simulink model "Model_Simscape_V2"  (R2023a)
settings: Solver=VariableStepAuto  StartTime=0.0  StopTime=10.0  RelTol=1e-3
model workspace (MAT data in the model file):
  Air_density = 1.29
  Body_Temperature = 37
  CtrlData_Max = 100
  CtrlData_Min = 0
  Detpress_to_Vavle.detpress = [1.45 1.55 1.6 1.65 1.7 1.75 1.8 1.85 1.9 1.95 2 2.05 5 7 26 42 60 78 99 112]
  Detpress_to_Vavle.vavle = [0.999 0.94 0.89 0.84 0.78 0.73 0.68 0.63 0.57 0.52 0.47 0.42 0.36 0.31 0.25 0.21 0.15 0.1 0.05 0]
  E_respriatory = 10
  ExpValve.opening_vector = [0 0.052 0.105 0.157 0.21 0.263 0.315 0.368 0.421 0.473 0.526 0.578 0.631 0.684 0.736 0.789 0.842 0.894 0.947 1]
  ExpValve.Cv_vector = [0.0001 0.81 1.114 1.723 3.218 3.547 4.603 5.2063 6.069 6.57 6.974 7.226 7.563 7.856 7.997 8.565 8.84 9.267 9.621 10.487]
  ExpValve.threshold = 0.0011
  ExpValve.zerovalue = 0
  ExpValve.Cross_Area = 0.000314159265359
  ExpValve.fullValue = 1
  FRC = 2
  Fan.shaftspeed = [14400 15600 16800 18000 19200 20400 21600 22800 24000 25200 26400 27600 28800 30000 31200 32400 33600 34800 36000 37200 38400 39600 40800 42000 43200 44400 45600 46800 48000]
  Fan.presstable = [0; 1; 2; 3; 4; 5; 6; 7; 8]
  Fan.flowvector = [97.5714285714 106 114 122 128.666666667 137 147.5 160.272727273 169.5 178.424242424 186.909090909 195.25 ... (261 elements, 29x9)]
  Fan.efficiency = [0.45  0.45  NaN  NaN  NaN  NaN  NaN  NaN  NaN; 0.45  0.45  NaN  NaN  NaN  NaN  NaN  NaN  NaN; 0.45  0.45  NaN  NaN  NaN  NaN  NaN  NaN  NaN; 0.45  0.45  NaN  NaN  NaN  NaN  NaN  NaN  NaN; 0.45  0.45  NaN  NaN  NaN  NaN  NaN  NaN  NaN; 0.45  0.45  NaN  NaN  NaN  NaN  NaN  NaN  NaN; 0.45  0.45  0.45  NaN  NaN  NaN  NaN  NaN  NaN; 0.45  0.45  0.45  NaN  NaN  NaN  NaN  NaN  NaN; 0.45  0.45  0.45  0.45  NaN  NaN  NaN  NaN  NaN; 0.45  0.45  0.45  0.45  NaN  NaN  NaN  NaN  NaN; 0.45  0.45  0.45  0.45  NaN  NaN  NaN  NaN  NaN; 0.45  0.45  0.45  0.45  NaN  NaN  NaN  NaN  NaN; 0.45  0.45  0.45  0.45  NaN  NaN  NaN  NaN  NaN; 0.45  0.45  0.45  0.45  0.45  NaN  NaN  NaN  NaN; 0.45  0.45  0.45  0.45  0.45  NaN  NaN  NaN  NaN; 0.45  0.45  0.45  0.45  0.45  NaN  NaN  NaN  NaN; 0.45  0.45  0.45  0.45  0.45  0.45  NaN  NaN  NaN; 0.45  0.45  0.45  0.45  0.45  0.45  NaN  NaN  NaN; 0.45  0.45  0.45  0.45  0.45  0.45  0.45  NaN  NaN; 0.45  0.45  0.45  0.45  0.45  0.45  0.45  NaN  NaN; 0.45  0.45  0.45  0.45  0.45  0.45  0.45  NaN  NaN; 0.45  0.45  0.45  0.45  0.45  0.45  0.45  NaN  NaN; 0.45  0.45  0.45  0.45  0.45  0.45  0.45  0.45  NaN; 0.45  0.45  0.45  0.45  0.45  0.45  0.45  0.45  NaN; 0.45  0.45  0.45  0.45  0.45  0.45  0.45  0.45  NaN; 0.45  0.45  0.45  0.45  0.45  0.45  0.45  0.45  0.45; 0.45  0.45  0.45  0.45  0.45  0.45  0.45  0.45  0.45; 0.45  0.45  0.45  0.45  0.45  0.45  0.45  0.45  0.45; 0.45  0.45  0.45  0.45  0.45  0.45  0.45  0.45  0.45]
  Fan.Inlerarea_A = 0.000314159265359
  Fan.Inlerarea_B = 0.000314159265359
  Flow_Resistance_1.resistance = 0.1
  Flow_Resistance_1.pressure_drop = 0.1
  Flow_Resistance_1.flow_rate = 1
  Flow_Resistance_1.Crosss_Area = 0.000314159265359
  Flow_Resistance_2.resistance = 0.1
  Flow_Resistance_2.pressure_drop = 0.1
  Flow_Resistance_2.flow_rate = 1
  Flow_Resistance_2.Crosss_Area = 0.000314159265359
  Hard_Stop.Lower_bound = -1e-06
  InspValve.opening_vector = [0 0.052 0.105 0.157 0.21 0.263 0.315 0.368 0.421 0.473 0.526 0.578 0.631 0.684 0.736 0.789 0.842 0.894 0.947 1]
  InspValve.Cv_vector = [0.0001 0.81 1.114 1.723 3.218 3.547 4.603 5.2063 6.069 6.57 6.974 7.226 7.563 7.856 7.997 8.565 8.84 9.267 9.621 10.487]
  InspValve.threshold = 0.0011
  InspValve.zerovalue = 0
  InspValve.Cross_Area = 0.000314159265359
  L_to_m3 = 0.001
  Mask.Chamber_volume = 0.0002
  Mask.A_area = 0.000314159265359
  Mask.B_area = 0.000314159265359
  Mask.C_area = 0.000314159265359
  Pa_to_cmH2O = 0.0101974428892
  Percent_to_Unit = 0.01
  Pipe_1.r = 0.01
  Pipe_1.longlength = 0.1
  Pipe_1.area = 0.000314159265359
  Pipe_1.diameter = 0.02
  Pipe_2.r = 0.01
  Pipe_2.longlength = 0.1
  Pipe_2.area = 0.000314159265359
  Pipe_2.diameter = 0.02
  Pipe_3.r = 0.01
  Pipe_3.longlength = 0.1
  Pipe_3.area = 0.000314159265359
  Pipe_3.diameter = 0.02
  R_respiratory = 2
  Reservoir.Cross_area = 0.000314159265359
  Trachea.Pipe_length = 0.15
  Trachea.area = 0.000314159265359
  Trachea.Hydraulic_diameter = 0.02
  Volume_Max = 0.9
  cmH2O_to_Pa = 98.0638
  cmH2O_to_kPa = 0.0981
  lung.Interface_area = 1
  lung.Dead_volume = 1e-06
  lung.Cross_area = 0.000314159265359
  percentage_to_rpm = 600
libraries: fl_lib x62, nesl_utility x13, SimscapeFluids_lib x3, aerolibatmos2 x1
(part 1 of 3)
settings Model: DataDictionary=MVEPP_DataDict.sldd  Creator=xuluyu  LastModifiedBy=xuluyu
settings OptimizationCC: UseDivisionForNetSlopeComputation=on

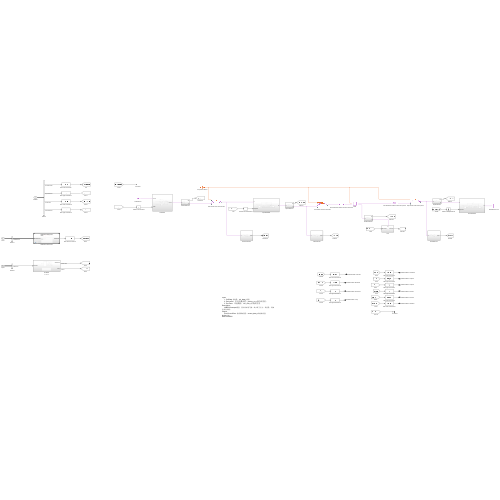
[thumbnail: Simulink's stored preview of the top-level diagram]
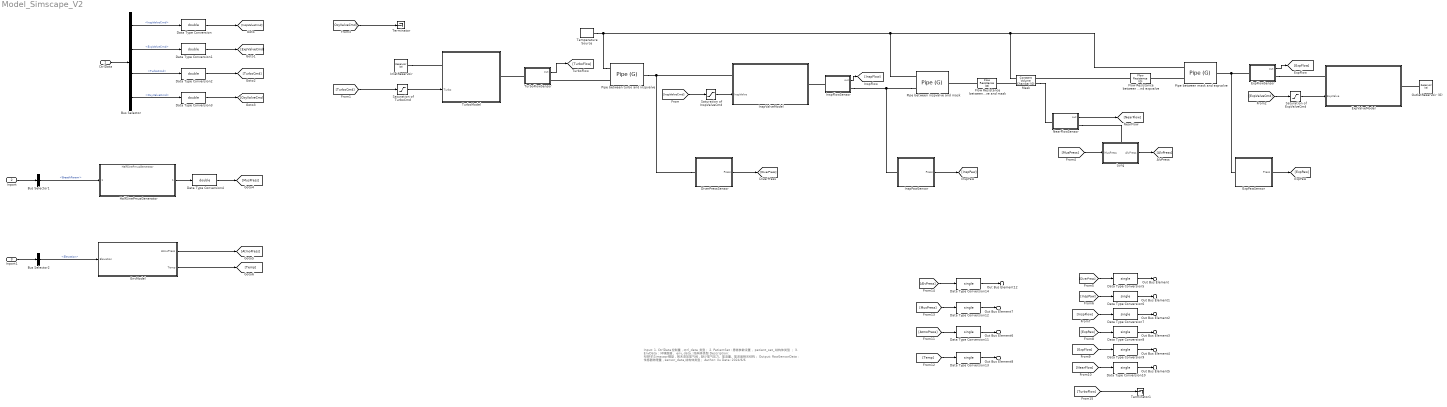
== system Model_Simscape_V2 ==
  note: Input:
      | 1. CtrlData: 控制量，ctrl_data_t类型；
      | 2. PatientSet ：患者参数设置， patient_set_t 结构体类型 ；
      | 3. EnvData ：环境数据， env_data_t 结构体类型
      | Description:
      | NIBP的Simscape模型，暂未添加氧气阀，缺少氧气压力、氧流量、氧浓度相关结构；
      | Output:
      | RawSensorData : 传感器物理量，sensor_data_t结构体类型；
      | Author: Xu
      | Data: 2024/6/6
  CtrlData : Inport  OutDataTypeStr=Bus: ctrl_data_t
  Inport : Inport  Port=2  OutDataTypeStr=Bus: patient_set_t
  Inport1 : Inport  Port=3  OutDataTypeStr=Bus: env_data_t
  Bus Selector : BusSelector  OutputSignals=InspValveCmd,ExpValveCmd,TurboCmd,OxyValveCmd
  Bus Selector1 : BusSelector  OutputSignals=BreathParam
  Bus Selector2 : BusSelector  OutputSignals=Elevation
  Data Type Conversion{,1..4} (5 alike) : DataTypeConversion  OutDataTypeStr=double  SaturateOnIntegerOverflow=off  RndMeth=Floor
  Data Type Conversion{5..14} (10 alike) : DataTypeConversion  OutDataTypeStr=single  SaturateOnIntegerOverflow=off  RndMeth=Floor
  DiverPressSensor : Subsystem
  EnvModel : Subsystem  Description=环境模型
      settings: AttributesFormatString=%<Description>
  ExpFlowSensor : Subsystem
  ExpPawSensor : Subsystem
  ExpValveModel : Subsystem
      settings: PortSchema="{\"entries\":[{\"content\":{\"sides\":[{\"content\":{\"connectorIds\":[\"LConn1\",\"In1\"]},\"type\":\"ConnectorPlacement.EquallySpacedRectSide\",\"uuid\":\"c1491169-4dad-48f4-8472-367eebf90c5f\"},{\"content\":{\"connectorIds\":[\"RConn1\"],\"side\":\"RIGHT\"},\"type\":\"ConnectorPlacement.EquallySpacedRectSide\",\"uuid\":\"0545f3b4-3593-4e73-91f2-3a40a520eda3\"},{\"content\":{\"side\":\"TOP\"},\"type\":\"ConnectorPlacement.EquallySpacedRectSide\",\"uuid\":\"424c4b06-b659-46bd-af11-3177a58fa4cf\"}]},\"type\":\"ConnectorPlacement.EquallySpacedConnector\",\"uuid\":\"6932a250-8b99-4db1-8a9b-8eee5e551d75\"}],\"packageUris\":[\"http://schema.mathworks.com/mf0/Connector/R2020b\"],\"version\":\"1.0\"}"
  Flow Resistance between inspvalve and mask : fl_lib/Gas/Elements/Flow Resistance (G)  delta_p_nominal=Flow_Resistance_1.pressure_drop*cmH2O_to_kPa kPa  mdot_nominal=Flow_Resistance_1.flow_rate*L_to_m3*Air_density kg/s  rho_nominal=0 kg/m^3  area=Flow_Resistance_1.Crosss_Area m^2  laminar_fraction=1e-3
      settings: InternalSimscapePortConfiguration="{\"Bottom\":[],\"Left\":[{\"id\":\"A\",\"label\":\"A\",\"type\":\"foundation.gas.gas\"}],\"Right\":[{\"id\":\"B\",\"label\":\"B\",\"type\":\"foundation.gas.gas\"}],\"Top\":[]}"
  Flow Resistance between mask and expvalve : fl_lib/Gas/Elements/Flow Resistance (G)  delta_p_nominal=Flow_Resistance_2.pressure_drop*cmH2O_to_kPa kPa  mdot_nominal=Flow_Resistance_2.flow_rate*L_to_m3*Air_density kg/s  rho_nominal=0 kg/m^3  area=Flow_Resistance_2.Crosss_Area m^2  laminar_fraction=1e-3
      settings: InternalSimscapePortConfiguration="{\"Bottom\":[],\"Left\":[{\"id\":\"A\",\"label\":\"A\",\"type\":\"foundation.gas.gas\"}],\"Right\":[{\"id\":\"B\",\"label\":\"B\",\"type\":\"foundation.gas.gas\"}],\"Top\":[]}"
  HalfSinePmusGenerator : ModelReference  ModelNameDialog=HalfSinePmusGenerator.slx  SimulationMode=Normal  ModelReferenceVersion=1.36
  InletReservoir : fl_lib/Gas/Elements/Reservoir (G)  pressure_spec=foundation.enum.pressure_spec.atmospheric  reservoir_pressure=0.101325 MPa  reservoir_temperature=293.15 K  area_A=Reservoir.Cross_area m^2
  "InspFlowSensor " : Subsystem
  InspPawSensor : Subsystem
  InspValveModel : Subsystem
      settings: PortSchema="{\"entries\":[{\"content\":{\"sides\":[{\"content\":{\"connectorIds\":[\"LConn1\",\"In1\"]},\"type\":\"ConnectorPlacement.EquallySpacedRectSide\",\"uuid\":\"c1491169-4dad-48f4-8472-367eebf90c5f\"},{\"content\":{\"connectorIds\":[\"RConn1\"],\"side\":\"RIGHT\"},\"type\":\"ConnectorPlacement.EquallySpacedRectSide\",\"uuid\":\"0545f3b4-3593-4e73-91f2-3a40a520eda3\"},{\"content\":{\"side\":\"TOP\"},\"type\":\"ConnectorPlacement.EquallySpacedRectSide\",\"uuid\":\"424c4b06-b659-46bd-af11-3177a58fa4cf\"}]},\"type\":\"ConnectorPlacement.EquallySpacedConnector\",\"uuid\":\"6932a250-8b99-4db1-8a9b-8eee5e551d75\"}],\"packageUris\":[\"http://schema.mathworks.com/mf0/Connector/R2020b\"],\"version\":\"1.0\"}"
  Lung : Subsystem
      settings: PortSchema="{\"entries\":[{\"content\":{\"sides\":[{\"content\":{\"connectorIds\":[\"In1\"]},\"type\":\"ConnectorPlacement.EquallySpacedRectSide\",\"uuid\":\"62194df3-39be-42c9-91e0-55317383e8ff\"},{\"content\":{\"connectorIds\":[\"Out1\"],\"side\":\"RIGHT\"},\"type\":\"ConnectorPlacement.EquallySpacedRectSide\",\"uuid\":\"0a91156d-be32-4862-8ff5-ef7fbd9fceb6\"},{\"content\":{\"connectorIds\":[\"LConn1\"],\"side\":\"TOP\"},\"type\":\"ConnectorPlacement.EquallySpacedRectSide\",\"uuid\":\"74941641-d695-41de-be65-3ac62a0b8891\"}]},\"type\":\"ConnectorPlacement.EquallySpacedConnector\",\"uuid\":\"a19a4056-8f95-4fbc-822a-a9438a1c1a7f\"}],\"packageUris\":[\"http://schema.mathworks.com/mf0/Connector/R2020b\"],\"version\":\"1.0\"}"
  Mask : fl_lib/Gas/Elements/Constant Volume Chamber (G)  volume=Mask.Chamber_volume m^3  num_ports=foundation.enum.num_ports.three  area_A=Mask.A_area m^2  area_B=Mask.B_area m^2  area_C=Mask.C_area m^2  area_D=0.01 m^2  p_I_specify=off  p_I_priority=High  p_I=0.101325 MPa  p_I_nominal_specify=off  p_I_nominal_unit=MPa  p_I_nominal_value=1  T_I_specify=off  T_I_priority=High  T_I=37 degC  T_I_nominal_specify=off  T_I_nominal_unit=K  T_I_nominal_value=1  rho_I_specify=off  rho_I_priority=None  rho_I=1.2 kg/m^3  rho_I_nominal_specify=off  rho_I_nominal_unit=kg/m^3  rho_I_nominal_value=1
      settings: InternalSimscapePortConfiguration="{\"Bottom\":[],\"Left\":[{\"id\":\"A\",\"label\":\"A\",\"type\":\"foundation.gas.gas\"},{\"id\":\"H\",\"label\":\"H\",\"type\":\"foundation.thermal.thermal\"}],\"Right\":[{\"id\":\"B\",\"label\":\"B\",\"type\":\"foundation.gas.gas\"},{\"id\":\"C\",\"label\":\"C\",\"type\":\"foundation.gas.gas\"}],\"Top\":[]}"
  "NearFlowSensor " : Subsystem
  OutletReservoir (G) : fl_lib/Gas/Elements/Reservoir (G)  pressure_spec=foundation.enum.pressure_spec.atmospheric  reservoir_pressure=0.101325 MPa  reservoir_temperature=293.15 K  area_A=Reservoir.Cross_area m^2
  Pipe between inspvalve and mask : fl_lib/Gas/Elements/Pipe (G)  length=Pipe_2.longlength m  area=Pipe_2.area m^2  Dh=Pipe_2.diameter m  length_add=0.1 m  roughness=15e-6 m  Re_lam=2000  Re_tur=4000  shape_factor=64  Nu_lam=3.66  p_I_specify=off  p_I_priority=High  p_I=0.101325 MPa  p_I_nominal_specify=off  p_I_nominal_unit=MPa  p_I_nominal_value=1  T_I_specify=off  T_I_priority=High  T_I=293.15 K  T_I_nominal_specify=off  T_I_nominal_unit=K  T_I_nominal_value=1  rho_I_specify=off  rho_I_priority=None  rho_I=1.2 kg/m^3  rho_I_nominal_specify=off  rho_I_nominal_unit=kg/m^3  rho_I_nominal_value=1
  Pipe between mask and expvalve : fl_lib/Gas/Elements/Pipe (G)  length=Pipe_3.longlength m  area=Pipe_3.area m^2  Dh=Pipe_3.diameter m  length_add=0.1 m  roughness=15e-6 m  Re_lam=2000  Re_tur=4000  shape_factor=64  Nu_lam=3.66  p_I_specify=off  p_I_priority=High  p_I=0.101325 MPa  p_I_nominal_specify=off  p_I_nominal_unit=MPa  p_I_nominal_value=1  T_I_specify=off  T_I_priority=High  T_I=293.15 K  T_I_nominal_specify=off  T_I_nominal_unit=K  T_I_nominal_value=1  rho_I_specify=off  rho_I_priority=None  rho_I=1.2 kg/m^3  rho_I_nominal_specify=off  rho_I_nominal_unit=kg/m^3  rho_I_nominal_value=1
  Pipe between turbo and inspvalve : fl_lib/Gas/Elements/Pipe (G)  length=Pipe_1.longlength m  area=Pipe_1.area m^2  Dh=Pipe_1.diameter m  length_add=0.1 m  roughness=15e-6 m  Re_lam=2000  Re_tur=4000  shape_factor=64  Nu_lam=3.66  p_I_specify=on  p_I_priority=High  p_I=0.101325 MPa  p_I_nominal_specify=off  p_I_nominal_unit=MPa  p_I_nominal_value=1  T_I_specify=on  T_I_priority=High  T_I=293.15 K  T_I_nominal_specify=off  T_I_nominal_unit=K  T_I_nominal_value=1  rho_I_specify=off  rho_I_priority=None  rho_I=1.2 kg/m^3  rho_I_nominal_specify=off  rho_I_nominal_unit=kg/m^3  rho_I_nominal_value=1
  Saturation of ExpValveCmd : Saturate  UpperLimit=CtrlData_Max  LowerLimit=CtrlData_Min
  Saturation of InspValveCmd : Saturate  UpperLimit=CtrlData_Max  LowerLimit=CtrlData_Min
  Saturation of TurboCmd : Saturate  UpperLimit=CtrlData_Max  LowerLimit=CtrlData_Min
  Temperature Source : fl_lib/Thermal/Thermal Sources/Temperature Source  temperature=293.15 K
  Terminator : Terminator
  Terminator1 : Terminator
  TurboFlowSensor : Subsystem
  TurboModel : Subsystem
      settings: PortSchema="{\"entries\":[{\"content\":{\"sides\":[{\"content\":{\"connectorIds\":[\"LConn1\",\"In1\"]},\"type\":\"ConnectorPlacement.EquallySpacedRectSide\",\"uuid\":\"c1491169-4dad-48f4-8472-367eebf90c5f\"},{\"content\":{\"connectorIds\":[\"RConn1\"],\"side\":\"RIGHT\"},\"type\":\"ConnectorPlacement.EquallySpacedRectSide\",\"uuid\":\"0545f3b4-3593-4e73-91f2-3a40a520eda3\"},{\"content\":{\"side\":\"TOP\"},\"type\":\"ConnectorPlacement.EquallySpacedRectSide\",\"uuid\":\"424c4b06-b659-46bd-af11-3177a58fa4cf\"}]},\"type\":\"ConnectorPlacement.EquallySpacedConnector\",\"uuid\":\"6932a250-8b99-4db1-8a9b-8eee5e551d75\"}],\"packageUris\":[\"http://schema.mathworks.com/mf0/Connector/R2020b\"],\"version\":\"1.0\"}"
  Out Bus Element6 : Outport  PortName=RawSensorData  Element=AtomPress
  Out Bus Element12 : Outport  PortName=RawSensorData  Element=AlvPress
  Out Bus Element7 : Outport  PortName=RawSensorData  Element=MusPress
  Out Bus Element2 : Outport  PortName=RawSensorData  Element=InspFlow
  Out Bus Element4 : Outport  PortName=RawSensorData  Element=ExpFlow
  Out Bus Element5 : Outport  PortName=RawSensorData  Element=NearFlow
  Out Bus Element1 : Outport  PortName=RawSensorData  Element=InspPaw
  Out Bus Element3 : Outport  PortName=RawSensorData  Element=ExpPaw
  Out Bus Element : Outport  PortName=RawSensorData  Element=DrivePress
  Out Bus Element8 : Outport  PortName=RawSensorData  Element=Temp
  wires:
  ExpFlowSensor/1(out) -> [ExpFlow]
  TurboFlowSensor/1(out) -> [TurboFlow]
  "NearFlowSensor "/1(out) -> [NearFlow]
  "InspFlowSensor "/1(out) -> [InspFlow]
  InspPawSensor/1(Press) -> [InspPaw]
  DiverPressSensor/1(Press) -> [DiverPress]
  ExpPawSensor/1(Press) -> [ExpPaw]
  CtrlData/1 -> Bus Selector/1
  Bus Selector/1 -> Data Type Conversion/1  "<InspValveCmd>"
  Bus Selector/2 -> Data Type Conversion1/1  "<ExpValveCmd>"
  Bus Selector/3 -> Data Type Conversion2/1  "<TurboCmd>"
  Bus Selector/4 -> Data Type Conversion3/1  "<OxyValveCmd>"
  Saturation of TurboCmd/1 -> TurboModel/1(Turbo)
  [TurboCmd] -> Saturation of TurboCmd/1
  Saturation of InspValveCmd/1 -> InspValveModel/1(InspValve)
  [InspValveCmd] -> Saturation of InspValveCmd/1
  [ExpValveCmd] -> Saturation of ExpValveCmd/1
  Saturation of ExpValveCmd/1 -> ExpValveModel/1(ExpValve)
  [OxyValveCmd] -> Terminator/1
  HalfSinePmusGenerator/1 -> Data Type Conversion4/1
  [MusPress] -> Lung/1(MusPress)
  Inport/1 -> Bus Selector1/1
  Bus Selector1/1 -> HalfSinePmusGenerator/1  "<BreathParam>"
  Data Type Conversion/1 -> [InspValveCmd]
  Data Type Conversion1/1 -> [ExpValveCmd]
  Data Type Conversion2/1 -> [TurboCmd]
  Data Type Conversion3/1 -> [OxyValveCmd]
  Data Type Conversion4/1 -> [MusPress]
  Inport1/1 -> Bus Selector2/1
  Bus Selector2/1 -> EnvModel/1(Elevation)  "<Elevation>"
  EnvModel/1(AtmoPress) -> [AtmoPress]
  EnvModel/2(Temp) -> [Temp]
  Lung/1(AlvPress) -> [AlvPress]
  [DiverPress] -> Data Type Conversion5/1
  [InspPaw] -> Data Type Conversion6/1
  [InspFlow] -> Data Type Conversion7/1
  [ExpPaw] -> Data Type Conversion8/1
  [ExpFlow] -> Data Type Conversion9/1
  [NearFlow] -> Data Type Conversion10/1
  [AtmoPress] -> Data Type Conversion11/1
  [MusPress] -> Data Type Conversion12/1
  [Temp] -> Data Type Conversion13/1
  Data Type Conversion5/1 -> Out Bus Element/1
  Data Type Conversion6/1 -> Out Bus Element1/1
  Data Type Conversion7/1 -> Out Bus Element2/1
  Data Type Conversion8/1 -> Out Bus Element3/1
  Data Type Conversion9/1 -> Out Bus Element4/1
  Data Type Conversion10/1 -> Out Bus Element5/1
  Data Type Conversion11/1 -> Out Bus Element6/1
  Data Type Conversion12/1 -> Out Bus Element7/1
  Data Type Conversion13/1 -> Out Bus Element8/1
  [AlvPress] -> Data Type Conversion14/1
  Data Type Conversion14/1 -> Out Bus Element12/1
  [TurboFlow] -> Terminator1/1
  connections:
  Pipe between mask and expvalve/RConn1 -- ExpFlowSensor/LConn1 -- ExpPawSensor/LConn1
  Pipe between inspvalve and mask/LConn1 -- "InspFlowSensor "/RConn1 -- InspPawSensor/LConn1
  DiverPressSensor/LConn1 -- InspValveModel/LConn1 -- Pipe between turbo and inspvalve/RConn1
  Pipe between turbo and inspvalve/LConn2 -- Pipe between mask and expvalve/LConn2 -- Mask/LConn2 -- Pipe between inspvalve and mask/LConn2 -- Temperature Source/LConn1
  Flow Resistance between inspvalve and mask/LConn1 -- Pipe between inspvalve and mask/RConn1
  "NearFlowSensor "/RConn1 -- Lung/LConn1
  Flow Resistance between mask and expvalve/LConn1 -- Mask/RConn2
  OutletReservoir (G)/LConn1 -- ExpValveModel/RConn1
  TurboFlowSensor/LConn1 -- TurboModel/RConn1
  ExpFlowSensor/RConn1 -- ExpValveModel/LConn1
  InletReservoir/LConn1 -- TurboModel/LConn1
  Mask/LConn1 -- Flow Resistance between inspvalve and mask/RConn1
  Pipe between turbo and inspvalve/LConn1 -- TurboFlowSensor/RConn1
  Mask/RConn1 -- "NearFlowSensor "/LConn1
  Pipe between mask and expvalve/LConn1 -- Flow Resistance between mask and expvalve/RConn1
  "InspFlowSensor "/LConn1 -- InspValveModel/RConn1

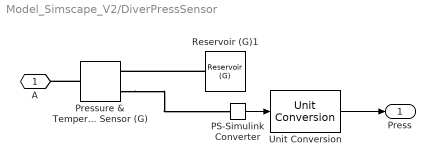
== system Model_Simscape_V2/DiverPressSensor ==
  PS-Simulink Converter : nesl_utility/PS-Simulink Converter  PhysicalDomain=network_engine_domain  SubClassName=ps_output  LeftPortType=input  RightPortType=output  PseudoPeriodic=off  Frequencies=[]  VectorFormat=inherit  Unit=Pa  AffineConversion=off
  Pressure & Temperature Sensor (G) : fl_lib/Gas/Sensors/Pressure & Temperature Sensor (G)  reference=foundation.enum.MeasurementReference.difference  pressure=true  pressure_spec=foundation.enum.PressureMeasementSpec.Absolute  temperature=false
      settings: InternalSimscapePortConfiguration="{\"Bottom\":[],\"Left\":[{\"id\":\"A\",\"label\":\"A\",\"type\":\"foundation.gas.gas\"}],\"Right\":[{\"id\":\"B\",\"label\":\"B\",\"type\":\"foundation.gas.gas\"},{\"id\":\"P\",\"label\":\"P\",\"type\":\"output\"}],\"Top\":[]}"
  Reservoir (G)1 : fl_lib/Gas/Elements/Reservoir (G)  pressure_spec=foundation.enum.pressure_spec.atmospheric  reservoir_pressure=0.101325 MPa  reservoir_temperature=293.15 K  area_A=Reservoir.Cross_area m^2
  Unit Conversion : UnitConversion
  A : PMIOPort  Side=Left
  Press : Outport  Unit=hPa
  wires:
  PS-Simulink Converter/1 -> Unit Conversion/1
  Unit Conversion/1 -> Press/1
  connections:
  Reservoir (G)1/LConn1 -- Pressure & Temperature Sensor (G)/RConn1
  Pressure & Temperature Sensor (G)/LConn1 -- A/RConn1
  Pressure & Temperature Sensor (G)/RConn2 -- PS-Simulink Converter/LConn1

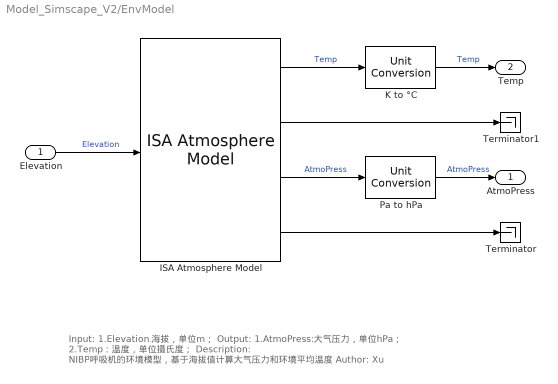
== system Model_Simscape_V2/EnvModel ==
  note: Input:
      | 	1.Elevation:海拔，单位m；
      | Output:
      | 	1.AtmoPress:大气压力，单位hPa；
      | 	2.Temp：温度，单位摄氏度；
      | Description:
      | 	NIBP呼吸机的环境模型，基于海拔值计算大气压力和环境平均温度
      | Author:
      | 	Xu
  Elevation : Inport  OutDataTypeStr=int16  Unit=m
  ISA Atmosphere Model : aerolibatmos2/ISA Atmosphere Model  custom=off  g=9.80665  gamma=1.4  R=287.0531  L=0.0065  h_trop=11000  h_strat=20000  rho0=1.225  P0=101325  T0=288.15  h0=0
  K to °C : UnitConversion  OutputType=Inherit: Inherit via back propagation
  Pa to hPa : UnitConversion  OutputType=Inherit: Inherit via back propagation
  Terminator : Terminator
  Terminator1 : Terminator
  AtmoPress : Outport  OutDataTypeStr=single  Unit=hPa
  Temp : Outport  Port=2  OutDataTypeStr=single  Unit=°C
  wires:
  Elevation/1 -> ISA Atmosphere Model/1  "Elevation"
  Pa to hPa/1 -> AtmoPress/1  "AtmoPress"
  ISA Atmosphere Model/4 -> Terminator/1
  K to °C/1 -> Temp/1  "Temp"
  ISA Atmosphere Model/2 -> Terminator1/1
  ISA Atmosphere Model/3 -> Pa to hPa/1  "AtmoPress"
  ISA Atmosphere Model/1 -> K to °C/1  "Temp"

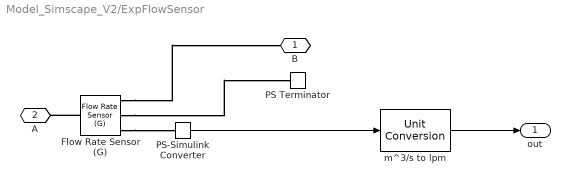
== system Model_Simscape_V2/ExpFlowSensor ==
  Flow Rate Sensor (G) : fl_lib/Gas/Sensors/Flow Rate Sensor (G)  mass_flow_measure=true  volumetric_flow_measure=true  volumetric_flow_conditions=foundation.enum.volumetric_flow_conditions.actual  p_std=0.101325 MPa  T_std=20 degC  energy_flow_measure=false
      settings: InternalSimscapePortConfiguration="{\"Bottom\":[],\"Left\":[{\"id\":\"A\",\"label\":\"A\",\"type\":\"foundation.gas.gas\"}],\"Right\":[{\"id\":\"B\",\"label\":\"B\",\"type\":\"foundation.gas.gas\"},{\"id\":\"M\",\"label\":\"M\",\"type\":\"output\"},{\"id\":\"V\",\"label\":\"V\",\"type\":\"output\"}],\"Top\":[]}"
  PS Terminator : fl_lib/Physical Signals/Sinks/PS Terminator
  PS-Simulink Converter : nesl_utility/PS-Simulink Converter  PhysicalDomain=network_engine_domain  SubClassName=ps_output  LeftPortType=input  RightPortType=output  PseudoPeriodic=off  Frequencies=[]  VectorFormat=inherit  Unit=m^3/s  AffineConversion=off
  m^3/s to lpm : UnitConversion
  B : PMIOPort  Side=Right
  A : PMIOPort  Port=2  Side=Left
  out : Outport  Unit=lpm
  wires:
  PS-Simulink Converter/1 -> m^3/s to lpm/1
  m^3/s to lpm/1 -> out/1
  connections:
  Flow Rate Sensor (G)/RConn1 -- B/RConn1
  Flow Rate Sensor (G)/LConn1 -- A/RConn1
  Flow Rate Sensor (G)/RConn2 -- PS Terminator/LConn1
  Flow Rate Sensor (G)/RConn3 -- PS-Simulink Converter/LConn1

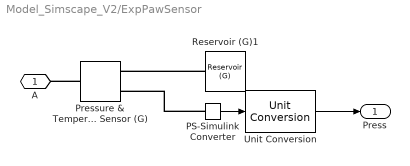
== system Model_Simscape_V2/ExpPawSensor ==
  PS-Simulink Converter : nesl_utility/PS-Simulink Converter  PhysicalDomain=network_engine_domain  SubClassName=ps_output  LeftPortType=input  RightPortType=output  PseudoPeriodic=off  Frequencies=[]  VectorFormat=inherit  Unit=inherit  AffineConversion=off
  Pressure & Temperature Sensor (G) : fl_lib/Gas/Sensors/Pressure & Temperature Sensor (G)  reference=foundation.enum.MeasurementReference.difference  pressure=true  pressure_spec=foundation.enum.PressureMeasementSpec.Absolute  temperature=false
      settings: InternalSimscapePortConfiguration="{\"Bottom\":[],\"Left\":[{\"id\":\"A\",\"label\":\"A\",\"type\":\"foundation.gas.gas\"}],\"Right\":[{\"id\":\"B\",\"label\":\"B\",\"type\":\"foundation.gas.gas\"},{\"id\":\"P\",\"label\":\"P\",\"type\":\"output\"}],\"Top\":[]}"
  Reservoir (G)1 : fl_lib/Gas/Elements/Reservoir (G)  pressure_spec=foundation.enum.pressure_spec.atmospheric  reservoir_pressure=0.101325 MPa  reservoir_temperature=293.15 K  area_A=Reservoir.Cross_area m^2
  Unit Conversion : UnitConversion
  A : PMIOPort  Side=Left
  Press : Outport  Unit=hPa
  wires:
  PS-Simulink Converter/1 -> Unit Conversion/1
  Unit Conversion/1 -> Press/1
  connections:
  PS-Simulink Converter/LConn1 -- Pressure & Temperature Sensor (G)/RConn2
  Reservoir (G)1/LConn1 -- Pressure & Temperature Sensor (G)/RConn1
  Pressure & Temperature Sensor (G)/LConn1 -- A/RConn1

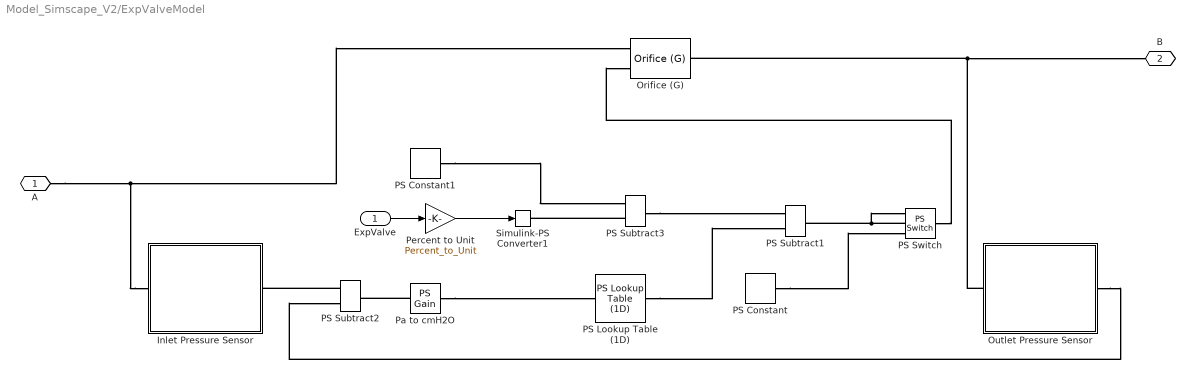
== system Model_Simscape_V2/ExpValveModel ==
  ExpValve : Inport
  " Inlet Pressure Sensor" : Subsystem
  " Outlet Pressure Sensor" : Subsystem
  Orifice (G) : SimscapeFluids_lib/Gas/Valves & Orifices/Orifice (G)  orifice_type=foundation.enum.constant_variable.variable  orifice_parameterization=fluids.gas.valves_orifices.enum.OrificeParameterization.Cv  opening_characteristic=fluids.gas.valves_orifices.enum.OpeningCharacteristics.Tabulated  Cv_constant=4  Cv_max=4  L_Cv_TLU=ExpValve.opening_vector  Cv_TLU=ExpValve.Cv_vector  xT_Cv=0.7  Kv_constant=3.6  Kv_max=3.6  L_Kv_TLU=0 : 0.2 : 1  Kv_TLU=[1e-06, .72, 1.44, 2.16, 2.88, 3.6]  xT_Kv=0.7  C_constant=12 l/(bar*s)  B_crit_constant=0.3  C_max=12 l/(bar*s)  B_crit_linear=0.3  L_C_TLU=0 : 0.2 : 1  C_TLU=[1e-05, 2.4, 4.8, 7.2, 9.6, 12] l/(bar*s)  B_crit_TLU=0.3 * ones(1, 6)  m=0.5  T_ref_C=293.15 K  rho_ref_C=1.185 kg/m^3  orifice_area_constant=1e-4 m^2  orifice_area_max=1e-4 m^2  L_orifice_area_TLU=0 : 0.2 : 1  orifice_area_TLU=[1e-10, 2e-05, 4e-05, 6e-05, 8e-05, .0001] m^2  Cd=0.64  leakage_fraction=1e-6  smoothing_factor=0.01  B_lam=0.999  area=ExpValve.Cross_Area m^2
      settings: InternalSimscapePortConfiguration="{\"Bottom\":[],\"Left\":[{\"id\":\"A\",\"label\":\"A\",\"type\":\"foundation.gas.gas\"},{\"id\":\"L\",\"label\":\"L\",\"type\":\"input\"}],\"Right\":[{\"id\":\"B\",\"label\":\"B\",\"type\":\"foundation.gas.gas\"}],\"Top\":[]}"
  PS Constant : fl_lib/Physical Signals/Sources/PS Constant  constant=ExpValve.zerovalue
  PS Constant1 : fl_lib/Physical Signals/Sources/PS Constant  constant=ExpValve.fullValue
  PS Lookup Table (1D) : fl_lib/Physical Signals/Lookup Tables/PS Lookup Table (1D)  x=Detpress_to_Vavle.detpress  f=Detpress_to_Vavle.vavle  interp_method=simscape.enum.interpolation.linear  extrap_method=simscape.enum.extrapolation.nearest
  PS Subtract1 : fl_lib/Physical Signals/Functions/PS Subtract
  PS Subtract2 : fl_lib/Physical Signals/Functions/PS Subtract
  PS Subtract3 : fl_lib/Physical Signals/Functions/PS Subtract
  PS Switch : fl_lib/Physical Signals/Nonlinear Operators/PS Switch  Threshold=ExpValve.threshold
      settings: InternalSimscapePortConfiguration="{\"Bottom\":[],\"Left\":[{\"id\":\"I1\",\"label\":\"\",\"type\":\"input\"},{\"id\":\"I2\",\"label\":\"\",\"type\":\"input\"},{\"id\":\"I3\",\"label\":\"\",\"type\":\"input\"}],\"Right\":[{\"id\":\"O\",\"label\":\"\",\"type\":\"output\"}],\"Top\":[]}"
  Pa to cmH2O : fl_lib/Physical Signals/Functions/PS Gain  gain=Pa_to_cmH2O 1/Pa
  Percent to Unit : Gain  Gain=Percent_to_Unit
  Simulink-PS Converter1 : nesl_utility/Simulink-PS Converter  PhysicalDomain=network_engine_domain  SubClassName=ps_input  LeftPortType=input  RightPortType=output  PseudoPeriodic=off  Frequencies=[]  NoiseDistribution=none  NoiseParameters=[]  Unit=1  AffineConversion=off  FilteringAndDerivatives=provide  SimscapeFilterOrder=1  InputFilterTimeConstant=0.001  UdotUserProvided=0
  A : PMIOPort  Side=Left
  B : PMIOPort  Port=2  Side=Right
  wires:
  Percent to Unit/1 -> Simulink-PS Converter1/1
  ExpValve/1 -> Percent to Unit/1
  connections:
  " Outlet Pressure Sensor"/LConn1 -- Orifice (G)/RConn1 -- B/RConn1
  PS Subtract2/LConn1 -- " Inlet Pressure Sensor"/RConn1
  PS Constant/RConn1 -- PS Switch/LConn3
  PS Switch/LConn2 -- PS Switch/LConn1 -- PS Subtract1/RConn1
  PS Lookup Table (1D)/RConn1 -- PS Subtract1/LConn2
  " Outlet Pressure Sensor"/RConn1 -- PS Subtract2/LConn2
  " Inlet Pressure Sensor"/LConn1 -- Orifice (G)/LConn1 -- A/RConn1
  PS Switch/RConn1 -- Orifice (G)/LConn2
  Pa to cmH2O/LConn1 -- PS Subtract2/RConn1
  Pa to cmH2O/RConn1 -- PS Lookup Table (1D)/LConn1
  PS Subtract3/LConn2 -- Simulink-PS Converter1/RConn1
  PS Subtract3/RConn1 -- PS Subtract1/LConn1
  PS Constant1/RConn1 -- PS Subtract3/LConn1

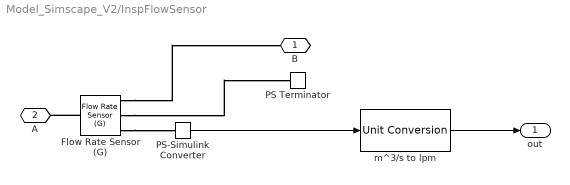
== system Model_Simscape_V2/InspFlowSensor  ==
  Flow Rate Sensor (G) : fl_lib/Gas/Sensors/Flow Rate Sensor (G)  mass_flow_measure=true  volumetric_flow_measure=true  volumetric_flow_conditions=foundation.enum.volumetric_flow_conditions.actual  p_std=0.101325 MPa  T_std=20 degC  energy_flow_measure=false
      settings: InternalSimscapePortConfiguration="{\"Bottom\":[],\"Left\":[{\"id\":\"A\",\"label\":\"A\",\"type\":\"foundation.gas.gas\"}],\"Right\":[{\"id\":\"B\",\"label\":\"B\",\"type\":\"foundation.gas.gas\"},{\"id\":\"M\",\"label\":\"M\",\"type\":\"output\"},{\"id\":\"V\",\"label\":\"V\",\"type\":\"output\"}],\"Top\":[]}"
  PS Terminator : fl_lib/Physical Signals/Sinks/PS Terminator
  PS-Simulink Converter : nesl_utility/PS-Simulink Converter  PhysicalDomain=network_engine_domain  SubClassName=ps_output  LeftPortType=input  RightPortType=output  PseudoPeriodic=off  Frequencies=[]  VectorFormat=inherit  Unit=m^3/s  AffineConversion=off
  m^3/s to lpm : UnitConversion
  B : PMIOPort  Side=Right
  A : PMIOPort  Port=2  Side=Left
  out : Outport  Unit=lpm
  wires:
  PS-Simulink Converter/1 -> m^3/s to lpm/1
  m^3/s to lpm/1 -> out/1
  connections:
  Flow Rate Sensor (G)/RConn1 -- B/RConn1
  Flow Rate Sensor (G)/LConn1 -- A/RConn1
  Flow Rate Sensor (G)/RConn2 -- PS Terminator/LConn1
  Flow Rate Sensor (G)/RConn3 -- PS-Simulink Converter/LConn1

== system Model_Simscape_V2/InspPawSensor ==
  PS-Simulink Converter : nesl_utility/PS-Simulink Converter  PhysicalDomain=network_engine_domain  SubClassName=ps_output  LeftPortType=input  RightPortType=output  PseudoPeriodic=off  Frequencies=[]  VectorFormat=inherit  Unit=inherit  AffineConversion=off
  Pressure & Temperature Sensor (G) : fl_lib/Gas/Sensors/Pressure & Temperature Sensor (G)  reference=foundation.enum.MeasurementReference.difference  pressure=true  pressure_spec=foundation.enum.PressureMeasementSpec.Absolute  temperature=false
      settings: InternalSimscapePortConfiguration="{\"Bottom\":[],\"Left\":[{\"id\":\"A\",\"label\":\"A\",\"type\":\"foundation.gas.gas\"}],\"Right\":[{\"id\":\"B\",\"label\":\"B\",\"type\":\"foundation.gas.gas\"},{\"id\":\"P\",\"label\":\"P\",\"type\":\"output\"}],\"Top\":[]}"
  Reservoir (G)1 : fl_lib/Gas/Elements/Reservoir (G)  pressure_spec=foundation.enum.pressure_spec.atmospheric  reservoir_pressure=0.101325 MPa  reservoir_temperature=293.15 K  area_A=Reservoir.Cross_area m^2
  Unit Conversion : UnitConversion
  A : PMIOPort  Side=Left
  Press : Outport  Unit=hPa
  wires:
  PS-Simulink Converter/1 -> Unit Conversion/1
  Unit Conversion/1 -> Press/1
  connections:
  Pressure & Temperature Sensor (G)/LConn1 -- A/RConn1
  Reservoir (G)1/LConn1 -- Pressure & Temperature Sensor (G)/RConn1
  PS-Simulink Converter/LConn1 -- Pressure & Temperature Sensor (G)/RConn2

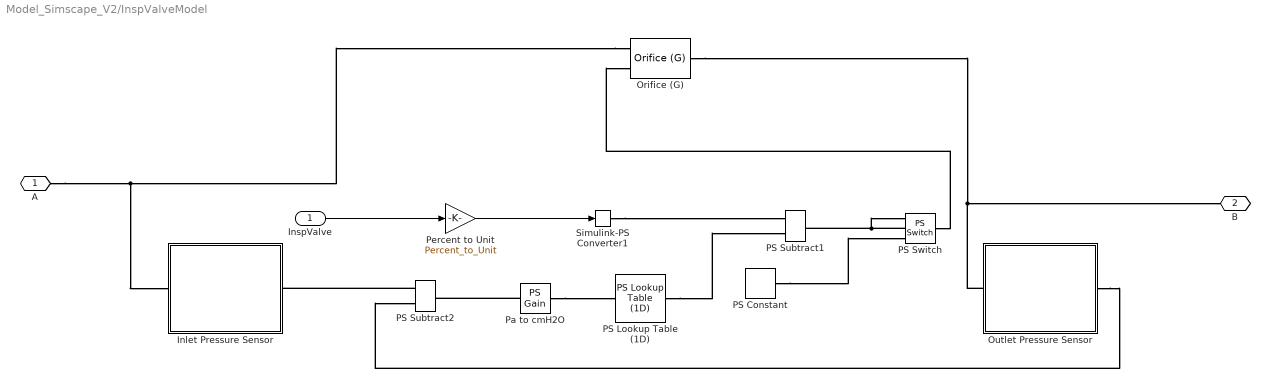
== system Model_Simscape_V2/InspValveModel ==
  InspValve : Inport
  " Inlet Pressure Sensor" : Subsystem
  " Outlet Pressure Sensor" : Subsystem
  Orifice (G) : SimscapeFluids_lib/Gas/Valves & Orifices/Orifice (G)  orifice_type=foundation.enum.constant_variable.variable  orifice_parameterization=fluids.gas.valves_orifices.enum.OrificeParameterization.Cv  opening_characteristic=fluids.gas.valves_orifices.enum.OpeningCharacteristics.Tabulated  Cv_constant=4  Cv_max=4  L_Cv_TLU=InspValve.opening_vector  Cv_TLU=InspValve.Cv_vector  xT_Cv=0.7  Kv_constant=3.6  Kv_max=3.6  L_Kv_TLU=0 : 0.2 : 1  Kv_TLU=[1e-06, .72, 1.44, 2.16, 2.88, 3.6]  xT_Kv=0.7  C_constant=12 l/(bar*s)  B_crit_constant=0.3  C_max=12 l/(bar*s)  B_crit_linear=0.3  L_C_TLU=0 : 0.2 : 1  C_TLU=[1e-05, 2.4, 4.8, 7.2, 9.6, 12] l/(bar*s)  B_crit_TLU=0.3 * ones(1, 6)  m=0.5  T_ref_C=293.15 K  rho_ref_C=1.185 kg/m^3  orifice_area_constant=1e-4 m^2  orifice_area_max=1e-4 m^2  L_orifice_area_TLU=0 : 0.2 : 1  orifice_area_TLU=[1e-10, 2e-05, 4e-05, 6e-05, 8e-05, .0001] m^2  Cd=0.64  leakage_fraction=1e-6  smoothing_factor=0.01  B_lam=0.999  area=InspValve.Cross_Area m^2
      settings: InternalSimscapePortConfiguration="{\"Bottom\":[],\"Left\":[{\"id\":\"A\",\"label\":\"A\",\"type\":\"foundation.gas.gas\"},{\"id\":\"L\",\"label\":\"L\",\"type\":\"input\"}],\"Right\":[{\"id\":\"B\",\"label\":\"B\",\"type\":\"foundation.gas.gas\"}],\"Top\":[]}"
  PS Constant : fl_lib/Physical Signals/Sources/PS Constant  constant=InspValve.zerovalue
  PS Lookup Table (1D) : fl_lib/Physical Signals/Lookup Tables/PS Lookup Table (1D)  x=Detpress_to_Vavle.detpress  f=Detpress_to_Vavle.vavle  interp_method=simscape.enum.interpolation.linear  extrap_method=simscape.enum.extrapolation.nearest
  PS Subtract1 : fl_lib/Physical Signals/Functions/PS Subtract
  PS Subtract2 : fl_lib/Physical Signals/Functions/PS Subtract
  PS Switch : fl_lib/Physical Signals/Nonlinear Operators/PS Switch  Threshold=InspValve.threshold
      settings: InternalSimscapePortConfiguration="{\"Bottom\":[],\"Left\":[{\"id\":\"I1\",\"label\":\"\",\"type\":\"input\"},{\"id\":\"I2\",\"label\":\"\",\"type\":\"input\"},{\"id\":\"I3\",\"label\":\"\",\"type\":\"input\"}],\"Right\":[{\"id\":\"O\",\"label\":\"\",\"type\":\"output\"}],\"Top\":[]}"
  Pa to cmH2O : fl_lib/Physical Signals/Functions/PS Gain  gain=Pa_to_cmH2O 1/Pa
  Percent to Unit : Gain  Gain=Percent_to_Unit
  Simulink-PS Converter1 : nesl_utility/Simulink-PS Converter  PhysicalDomain=network_engine_domain  SubClassName=ps_input  LeftPortType=input  RightPortType=output  PseudoPeriodic=off  Frequencies=[]  NoiseDistribution=none  NoiseParameters=[]  Unit=1  AffineConversion=off  FilteringAndDerivatives=provide  SimscapeFilterOrder=1  InputFilterTimeConstant=0.001  UdotUserProvided=0
  A : PMIOPort  Side=Left
  B : PMIOPort  Port=2  Side=Right
  wires:
  InspValve/1 -> Percent to Unit/1
  Percent to Unit/1 -> Simulink-PS Converter1/1
  connections:
  Orifice (G)/RConn1 -- " Outlet Pressure Sensor"/LConn1 -- B/RConn1
  PS Subtract2/LConn1 -- " Inlet Pressure Sensor"/RConn1
  PS Constant/RConn1 -- PS Switch/LConn3
  PS Switch/LConn2 -- PS Subtract1/RConn1 -- PS Switch/LConn1
  PS Lookup Table (1D)/RConn1 -- PS Subtract1/LConn2
  " Outlet Pressure Sensor"/RConn1 -- PS Subtract2/LConn2
  Orifice (G)/LConn1 -- A/RConn1 -- " Inlet Pressure Sensor"/LConn1
  Simulink-PS Converter1/RConn1 -- PS Subtract1/LConn1
  PS Switch/RConn1 -- Orifice (G)/LConn2
  Pa to cmH2O/LConn1 -- PS Subtract2/RConn1
  Pa to cmH2O/RConn1 -- PS Lookup Table (1D)/LConn1

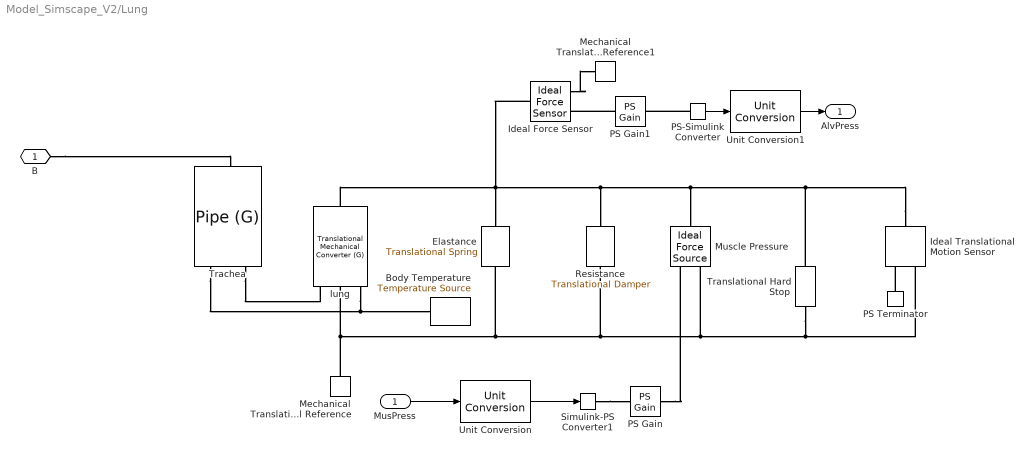
== system Model_Simscape_V2/Lung ==
  MusPress : Inport  Unit=hPa
  Body Temperature : fl_lib/Thermal/Thermal Sources/Temperature Source  temperature="Body_Temperature  degC"
  Elastance : fl_lib/Mechanical/Translational Elements/Translational Spring  spr_rate=E_respriatory*(lung.Interface_area^2)*(cmH2O_to_Pa/L_to_m3) N/m  v_specify=off  v_priority=None  v=0 m/s  v_nominal_specify=off  v_nominal_unit=m/s  v_nominal_value=1  f_specify=off  f_priority=None  f=0 N  f_nominal_specify=off  f_nominal_unit=N  f_nominal_value=1  x_specify=off  x_priority=High  x=0 m  x_nominal_specify=off  x_nominal_unit=m  x_nominal_value=1
  Ideal Force Sensor : fl_lib/Mechanical/Mechanical Sensors/Ideal Force Sensor
  Ideal Translational Motion Sensor : fl_lib/Mechanical/Mechanical Sensors/Ideal Translational Motion Sensor  reference=foundation.enum.MeasurementReference.difference  acceleration_port=false  velocity_port=false  position_port=true  offset=FRC*L_to_m3 m
      settings: InternalSimscapePortConfiguration="{\"Bottom\":[],\"Left\":[{\"id\":\"R\",\"label\":\"R\",\"type\":\"foundation.mechanical.translational.translational\"}],\"Right\":[{\"id\":\"C\",\"label\":\"C\",\"type\":\"foundation.mechanical.translational.translational\"},{\"id\":\"P\",\"label\":\"P\",\"type\":\"output\"}],\"Top\":[]}"
  Mechanical Translational Reference : fl_lib/Mechanical/Translational Elements/Mechanical Translational Reference
  Mechanical Translational Reference1 : fl_lib/Mechanical/Translational Elements/Mechanical Translational Reference
  Muscle Pressure : fl_lib/Mechanical/Mechanical Sources/Ideal Force Source
  PS Gain : fl_lib/Physical Signals/Functions/PS Gain  gain=lung.Interface_area m^2
  PS Gain1 : fl_lib/Physical Signals/Functions/PS Gain  gain=1/lung.Interface_area 1/m^2
  PS Terminator : fl_lib/Physical Signals/Sinks/PS Terminator
  PS-Simulink Converter : nesl_utility/PS-Simulink Converter  PhysicalDomain=network_engine_domain  SubClassName=ps_output  LeftPortType=input  RightPortType=output  PseudoPeriodic=off  Frequencies=[]  VectorFormat=inherit  Unit=Pa  AffineConversion=off
  Resistance : fl_lib/Mechanical/Translational Elements/Translational Damper  D=R_respiratory*(lung.Interface_area^2)*(cmH2O_to_Pa/L_to_m3) N*s/m  v_specify=off  v_priority=None  v=0 m/s  v_nominal_specify=off  v_nominal_unit=m/s  v_nominal_value=1  f_specify=off  f_priority=None  f=0 N  f_nominal_specify=off  f_nominal_unit=N  f_nominal_value=1
  Simulink-PS Converter1 : nesl_utility/Simulink-PS Converter  PhysicalDomain=network_engine_domain  SubClassName=ps_input  LeftPortType=input  RightPortType=output  PseudoPeriodic=off  Frequencies=[]  NoiseDistribution=none  NoiseParameters=[]  Unit=Pa  AffineConversion=off  FilteringAndDerivatives=provide  SimscapeFilterOrder=1  InputFilterTimeConstant=0.001  UdotUserProvided=0
  Trachea : fl_lib/Gas/Elements/Pipe (G)  length=Trachea.Pipe_length m  area=Trachea.area m^2  Dh=Trachea.Hydraulic_diameter m  length_add=0.1 m  roughness=15e-6 m  Re_lam=2000  Re_tur=4000  shape_factor=64  Nu_lam=3.66  p_I_specify=off  p_I_priority=High  p_I=0.101325 MPa  p_I_nominal_specify=off  p_I_nominal_unit=MPa  p_I_nominal_value=1  T_I_specify=on  T_I_priority=High  T_I=37 degC  T_I_nominal_specify=off  T_I_nominal_unit=K  T_I_nominal_value=1  rho_I_specify=off  rho_I_priority=None  rho_I=1.2 kg/m^3  rho_I_nominal_specify=off  rho_I_nominal_unit=kg/m^3  rho_I_nominal_value=1
  Translational Hard Stop : fl_lib/Mechanical/Translational Elements/Translational Hard Stop  upper_bnd=Volume_Max*L_to_m3/lung.Interface_area m  lower_bnd=Hard_Stop.Lower_bound m  model=simscape.enum.hardstop.modechart  stiff_up=1e6 N/m  stiff_low=1e6 N/m  D_up=350 N*s/m  D_low=350 N*s/m  transition=0.01 mm  coeff_rest=0.7  v_tol=0.001 m/s  f_tol=0.001 N  x_specify=off  x_priority=High  x=lung.Initial_displacement m  x_nominal_specify=off  x_nominal_unit=m  x_nominal_value=1  v_specify=off  v_priority=None  v=0 m/s  v_nominal_specify=off  v_nominal_unit=m/s  v_nominal_value=1  f_specify=off  f_priority=None  f=0 N  f_nominal_specify=off  f_nominal_unit=N  f_nominal_value=1  M_specify=off  M_priority=None  M=0
  Unit Conversion : UnitConversion
  Unit Conversion1 : UnitConversion
  lung : fl_lib/Gas/Elements/Translational Mechanical Converter (G)  mech_orientation=foundation.enum.MechOrientationTranslational.Positive  displacement_spec=foundation.enum.DisplacementSpec.Calculate  length_init=FRC*L_to_m3 m  interface_area=lung.Interface_area m^2  dead_volume=lung.Dead_volume m^3  area_A=lung.Cross_area m^2  environment_spec=foundation.enum.pressure_spec.atmospheric  environment_pressure=0.101325 MPa  p_I_specify=off  p_I_priority=High  p_I=0.101325 MPa  p_I_nominal_specify=off  p_I_nominal_unit=MPa  p_I_nominal_value=1  T_I_specify=on  T_I_priority=High  T_I="Body_Temperature  degC"  T_I_nominal_specify=off  T_I_nominal_unit=K  T_I_nominal_value=1  rho_I_specify=off  rho_I_priority=None  rho_I=1.2 kg/m^3  rho_I_nominal_specify=off  rho_I_nominal_unit=kg/m^3  rho_I_nominal_value=1
      settings: InternalSimscapePortConfiguration="{\"Bottom\":[],\"Left\":[{\"id\":\"A\",\"label\":\"A\",\"type\":\"foundation.gas.gas\"},{\"id\":\"C\",\"label\":\"C\",\"type\":\"foundation.mechanical.translational.translational\"},{\"id\":\"H\",\"label\":\"H\",\"type\":\"foundation.thermal.thermal\"}],\"Right\":[{\"id\":\"R\",\"label\":\"R\",\"type\":\"foundation.mechanical.translational.translational\"}],\"Top\":[]}"
  B : PMIOPort  Side=Left
  AlvPress : Outport  Unit=hPa
  wires:
  MusPress/1 -> Unit Conversion/1
  Unit Conversion/1 -> Simulink-PS Converter1/1
  PS-Simulink Converter/1 -> Unit Conversion1/1
  Unit Conversion1/1 -> AlvPress/1
  connections:
  Trachea/LConn1 -- lung/LConn1
  Resistance/RConn1 -- Mechanical Translational Reference/LConn1 -- lung/LConn2 -- Elastance/RConn1 -- Translational Hard Stop/RConn1 -- Ideal Translational Motion Sensor/RConn1 -- Muscle Pressure/RConn2
  Ideal Translational Motion Sensor/LConn1 -- Elastance/LConn1 -- Ideal Force Sensor/LConn1 -- lung/RConn1 -- Resistance/LConn1 -- Muscle Pressure/LConn1 -- Translational Hard Stop/LConn1
  PS Terminator/LConn1 -- Ideal Translational Motion Sensor/RConn2
  Trachea/LConn2 -- lung/LConn3 -- Body Temperature/LConn1
  B/RConn1 -- Trachea/RConn1
  Simulink-PS Converter1/RConn1 -- PS Gain/LConn1
  PS Gain/RConn1 -- Muscle Pressure/RConn1
  PS Gain1/LConn1 -- Ideal Force Sensor/RConn2
  Ideal Force Sensor/RConn1 -- Mechanical Translational Reference1/LConn1
  PS-Simulink Converter/LConn1 -- PS Gain1/RConn1

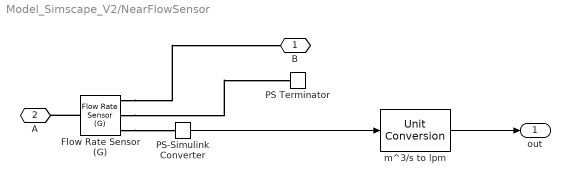
== system Model_Simscape_V2/NearFlowSensor  ==
  Flow Rate Sensor (G) : fl_lib/Gas/Sensors/Flow Rate Sensor (G)  mass_flow_measure=true  volumetric_flow_measure=true  volumetric_flow_conditions=foundation.enum.volumetric_flow_conditions.actual  p_std=0.101325 MPa  T_std=20 degC  energy_flow_measure=false
      settings: InternalSimscapePortConfiguration="{\"Bottom\":[],\"Left\":[{\"id\":\"A\",\"label\":\"A\",\"type\":\"foundation.gas.gas\"}],\"Right\":[{\"id\":\"B\",\"label\":\"B\",\"type\":\"foundation.gas.gas\"},{\"id\":\"M\",\"label\":\"M\",\"type\":\"output\"},{\"id\":\"V\",\"label\":\"V\",\"type\":\"output\"}],\"Top\":[]}"
  PS Terminator : fl_lib/Physical Signals/Sinks/PS Terminator
  PS-Simulink Converter : nesl_utility/PS-Simulink Converter  PhysicalDomain=network_engine_domain  SubClassName=ps_output  LeftPortType=input  RightPortType=output  PseudoPeriodic=off  Frequencies=[]  VectorFormat=inherit  Unit=m^3/s  AffineConversion=off
  m^3/s to lpm : UnitConversion
  B : PMIOPort  Side=Right
  A : PMIOPort  Port=2  Side=Left
  out : Outport  Unit=lpm
  wires:
  m^3/s to lpm/1 -> out/1
  PS-Simulink Converter/1 -> m^3/s to lpm/1
  connections:
  Flow Rate Sensor (G)/RConn3 -- PS-Simulink Converter/LConn1
  Flow Rate Sensor (G)/RConn2 -- PS Terminator/LConn1
  Flow Rate Sensor (G)/LConn1 -- A/RConn1
  Flow Rate Sensor (G)/RConn1 -- B/RConn1

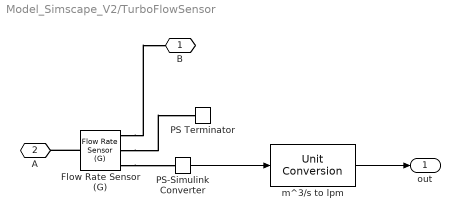
== system Model_Simscape_V2/TurboFlowSensor ==
  Flow Rate Sensor (G) : fl_lib/Gas/Sensors/Flow Rate Sensor (G)  mass_flow_measure=true  volumetric_flow_measure=true  volumetric_flow_conditions=foundation.enum.volumetric_flow_conditions.actual  p_std=0.101325 MPa  T_std=20 degC  energy_flow_measure=false
      settings: InternalSimscapePortConfiguration="{\"Bottom\":[],\"Left\":[{\"id\":\"A\",\"label\":\"A\",\"type\":\"foundation.gas.gas\"}],\"Right\":[{\"id\":\"B\",\"label\":\"B\",\"type\":\"foundation.gas.gas\"},{\"id\":\"M\",\"label\":\"M\",\"type\":\"output\"},{\"id\":\"V\",\"label\":\"V\",\"type\":\"output\"}],\"Top\":[]}"
  PS Terminator : fl_lib/Physical Signals/Sinks/PS Terminator
  PS-Simulink Converter : nesl_utility/PS-Simulink Converter  PhysicalDomain=network_engine_domain  SubClassName=ps_output  LeftPortType=input  RightPortType=output  PseudoPeriodic=off  Frequencies=[]  VectorFormat=inherit  Unit=m^3/s  AffineConversion=off
  m^3/s to lpm : UnitConversion
  B : PMIOPort  Side=Right
  A : PMIOPort  Port=2  Side=Left
  out : Outport  Unit=lpm
  wires:
  m^3/s to lpm/1 -> out/1
  PS-Simulink Converter/1 -> m^3/s to lpm/1
  connections:
  Flow Rate Sensor (G)/RConn3 -- PS-Simulink Converter/LConn1
  Flow Rate Sensor (G)/RConn2 -- PS Terminator/LConn1
  Flow Rate Sensor (G)/LConn1 -- A/RConn1
  Flow Rate Sensor (G)/RConn1 -- B/RConn1
